simulink model "sin_spectrum"  (R2024a)
settings: Solver=VariableStepAuto  StartTime=0.0  StopTime=10.0  RelTol=1e-3
settings Model: Creator=evgenijkondratev  LastModifiedBy=evgenijkondratev

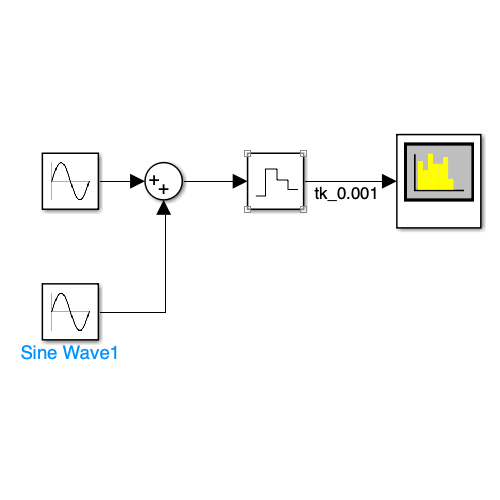
[thumbnail: Simulink's stored preview of the top-level diagram]
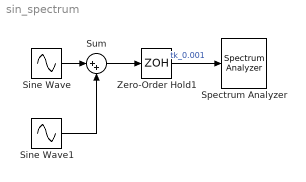
== system sin_spectrum ==
  Sine Wave : Sin  Frequency=100  SampleTime=0
  Sine Wave1 : Sin  Amplitude=2  Frequency=50  SampleTime=0
  Spectrum Analyzer : SpectrumAnalyzer  WindowPosition=[560.000000,290.000000,800.000000,500.000000,]  ScopeFrameLocation=window  Span=1000  StartFrequency=-500  StopFrequency=500  YLimits=[21.717807013416994,29.53191934956406]
  Sum : Sum  Inputs=|++
  Zero-Order Hold1 : ZeroOrderHold  SampleTime=0.001
  wires:
  Zero-Order Hold1/1 -> Spectrum Analyzer/1  "tk_0.001"
  Sine Wave/1 -> Sum/1
  Sine Wave1/1 -> Sum/2
  Sum/1 -> Zero-Order Hold1/1
